simulink model "Outer1"  (Simulink 8.7)
settings: Solver=ode45  StartTime=0.0  StopTime=10.0  RelTol=1e-3
settings Model: Creator=scaife  LastModifiedBy=bourbouh  ExtModeAutoUpdateStatusClock=off
settings DataIOCC: SignalLoggingSaveFormat=ModelDataLogs  SignalLoggingName=sigsOut
settings DebuggingCC: SaveWithParameterizedLinksMsg=none  SignalResolutionControl=TryResolveAllWithWarning  MultiTaskDSMMsg=warning  MultiTaskCondExecSysMsg=none
settings HardwareCC: TargetUnknown=on
settings SFSimCC: SimParseCustomCode=off
settings GRTTargetCC: GeneratePreprocessorConditionals=Use local settings  CombineOutputUpdateFcns=off  GRTInterface=on

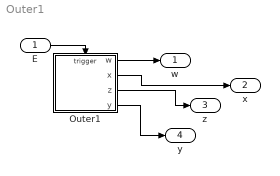
== system Outer1 ==
  E : Inport
  Outer1 : Stateflow chart  TreatAsAtomicUnit=on
  w : Outport
  x : Outport  Port=2
  z : Outport  Port=3
  y : Outport  Port=4
  wires:
  Outer1/1(w) -> w/1
  Outer1/2(x) -> x/1
  Outer1/3(z) -> z/1
  Outer1/4(y) -> y/1
  E/1 -> Outer1/Trigger

== stateflow chart Outer1 ==
  state A/
    en: z++;
    ex: w++;
  A -> A : E{x++;}/y++;
  (default) -> A
  data: w output int32; x output int32; z output int32; y output int32
  events: E input EITHER_EDGE_EVENT
